simulink model "MdXX_QuitReason"  (R2018b)
settings: Solver=FixedStepDiscrete  StartTime=0.0  StopTime=10.0  FixedStep=0.01  RelTol=1e-3
undefined symbols (not defined in the file or in its folder): MdRspLocal2
settings Model: Creator=sn2xws  LastModifiedBy=sn2xws
settings Model: ModifiedHistory=|
  | 2024.12.11 V3.0.0 CR955881
  | 2025.2.24 V3.0.1 BUG 9932326 将前提条件不满足的优先级提到最高
settings DataIOCC: SaveFormat=StructureWithTime
settings OptimizationCC: DefaultParameterBehavior=Inlined  EnhancedBackFolding=on  PassReuseOutputArgsAs=Individual arguments  ZeroExternalMemoryAtStartup=off  ZeroInternalMemoryAtStartup=off  OptimizeBlockOrder=speed  DifferentSizesBufferReuse=on  OptimizationCustomize=off
settings DebuggingCC: ParameterTunabilityLossMsg=error
settings SFSimCC: MATLABDynamicMemAlloc=off
settings RTWCC: SystemTargetFile=autosar.tlc  GenCodeOnly=on  TemplateMakefile=ert_default_tmf  Description=AUTOSAR  GenerateReport=on  IncludeHyperlinkInReport=on  LaunchReport=on  GenerateTraceInfo=on  GenerateTraceReport=on  GenerateTraceReportSl=on  GenerateTraceReportSf=on  GenerateTraceReportEml=on  GenerateCodeMetricsReport=on
settings CodeAppCC: ForceParamTrailComments=on  IgnoreCustomStorageClasses=off  OperatorAnnotations=on  SimulinkDataObjDesc=on  SFDataObjDesc=on  InsertBlockDesc=on
settings STFCustomTargetCC: TargetLangStandard=C99 (ISO)  MultiwordLength=256  ParMdlRefBuildCompliant=on  CompOptLevelCompliant=on  IncludeMdlTerminateFcn=off  CombineOutputUpdateFcns=on  SuppressErrorStatus=on  ERTCustomFileBanners=on  SupportNonFinite=off  SupportComplex=off  SupportContinuousTime=off  SupportNonInlinedSFcns=off  RemoveResetFunc=on  MATLABClassNameForMDSCustomization=Simulink.SoftwareTarget.ERTCustomization  AutosarCompliant=on  UseToolchainInfoCompliant=on  LookupTableObjectStructAxisOrder=2,1,3,4,...  LUTObjectStructOrderEvenSpacing=Size,Table,Breakpoints  SystemTargetFile=autosar.tlc
settings ERTTargetCC: TargetLangStandard=C99 (ISO)  ConcurrentExecutionCompliant=off  IncludeMdlTerminateFcn=off  SuppressErrorStatus=on  SupportNonFinite=off  SupportComplex=off  ModelStepFunctionPrototypeControlCompliant=off  CPPClassGenCompliant=off  AutosarCompliant=on  LookupTableObjectStructAxisOrder=2,1,3,4,...  LUTObjectStructOrderEvenSpacing=Size,Table,Breakpoints  InlinedParameterPlacement=NonHierarchical  ERTCustomFileTemplate=example_file_process.tlc  ERTFilePackagingFormat=Compact

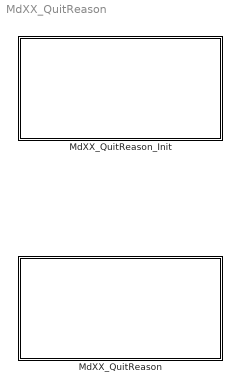
== system MdXX_QuitReason ==
  MdXX_QuitReason : Subsystem
  MdXX_QuitReason_Init : Subsystem

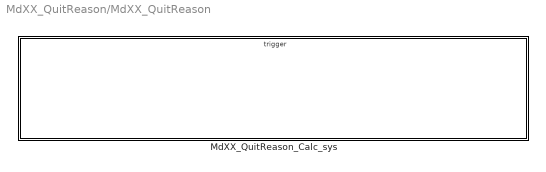
== system MdXX_QuitReason/MdXX_QuitReason ==
  MdXX_QuitReason_Calc_sys : Subsystem

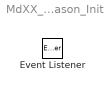
== system MdXX_QuitReason/MdXX_QuitReason_Init ==
  Event Listener : EventListener  EventName=reset

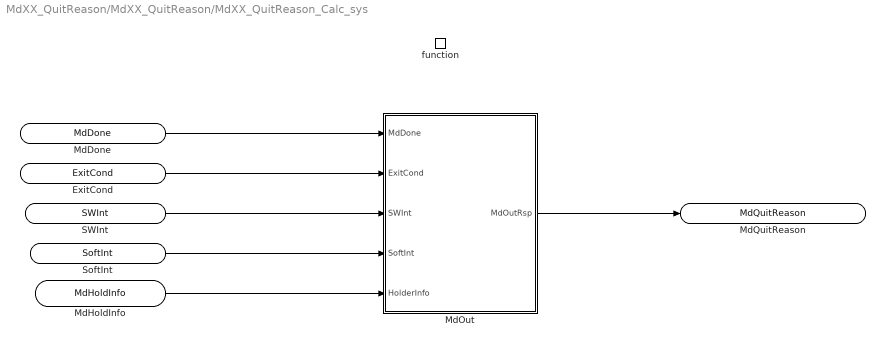
== system MdXX_QuitReason/MdXX_QuitReason/MdXX_QuitReason_Calc_sys ==
  function : TriggerPort  TriggerType=function-call  IsSimulinkFunction=on  FunctionName=MdXX_QuitReason_Calc  VariantControl=(inherit)
  MdOut : Subsystem  TreatAsAtomicUnit=on  RTWFcnName=MdRspChk
      settings: RTWFcnNameOpts=User specified
  MdDone : ArgIn  OutDataTypeStr=uint8  ArgumentName=MdDone
  ExitCond : ArgIn  Port=2  OutDataTypeStr=boolean  ArgumentName=ExitCond
  SWInt : ArgIn  Port=3  OutDataTypeStr=boolean  ArgumentName=SWInt
  SoftInt : ArgIn  Port=4  OutDataTypeStr=boolean  ArgumentName=SoftInt
  MdHoldInfo : ArgIn  Port=5  OutDataTypeStr=boolean  ArgumentName=MdHoldInfo
  MdQuitReason : ArgOut  OutDataTypeStr=Enum: MdRspLocal2  ArgumentName=MdQuitReason
  wires:
  MdDone/1 -> MdOut/1(MdDone)
  ExitCond/1 -> MdOut/2(ExitCond)
  SWInt/1 -> MdOut/3(SWInt)
  SoftInt/1 -> MdOut/4(SoftInt)
  MdOut/1(MdOutRsp) -> MdQuitReason/1
  MdHoldInfo/1 -> MdOut/5(HolderInfo)

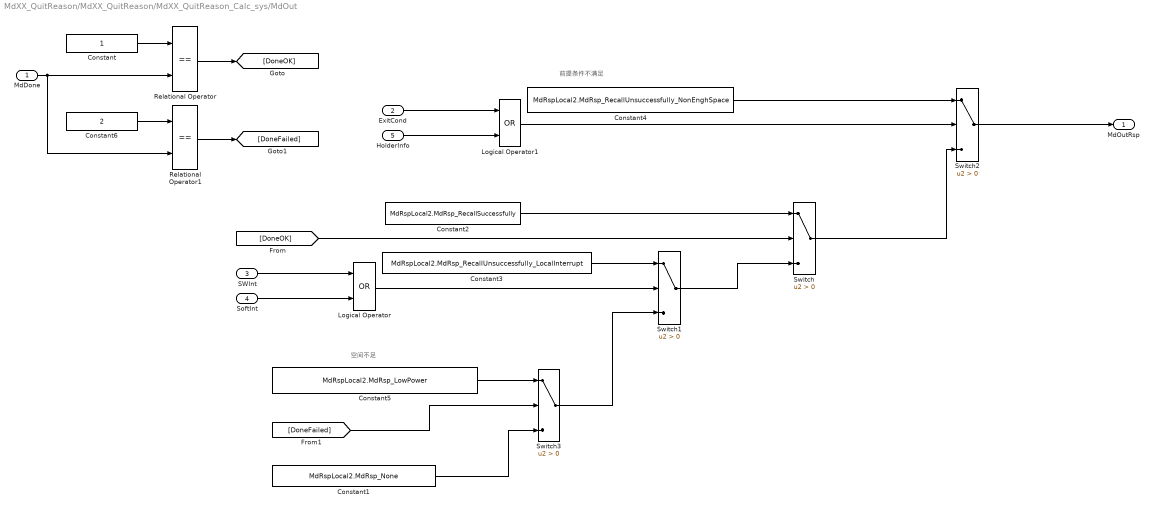
== system MdXX_QuitReason/MdXX_QuitReason/MdXX_QuitReason_Calc_sys/MdOut ==
  note: 前提条件不满足
  note: 空间不足
  MdDone : Inport
  ExitCond : Inport  Port=2
  SWInt : Inport  Port=3
  SoftInt : Inport  Port=4
  HolderInfo : Inport  Port=5
  Constant : Constant
  Constant1 : Constant  Value=MdRspLocal2.MdRsp_None  OutDataTypeStr=Enum:MdRspLocal2
  Constant2 : Constant  Value=MdRspLocal2.MdRsp_RecallSuccessfully  OutDataTypeStr=Enum:MdRspLocal2
  Constant3 : Constant  Value=MdRspLocal2.MdRsp_RecallUnsuccessfully_LocalInterrupt  OutDataTypeStr=Enum:MdRspLocal2
  Constant4 : Constant  Value=MdRspLocal2.MdRsp_RecallUnsuccessfully_NonEnghSpace  OutDataTypeStr=Enum:MdRspLocal2
  Constant5 : Constant  Value=MdRspLocal2.MdRsp_LowPower  OutDataTypeStr=Enum:MdRspLocal2
  Constant6 : Constant  Value=2
  Logical Operator : Logic  Operator=OR  AllPortsSameDT=off  OutDataTypeStr=boolean
  Logical Operator1 : Logic  Operator=OR  AllPortsSameDT=off  OutDataTypeStr=boolean
  Relational Operator : RelationalOperator  Operator===  OutDataTypeStr=boolean  RndMeth=Simplest
  Relational Operator1 : RelationalOperator  Operator===  OutDataTypeStr=boolean  RndMeth=Simplest
  Switch{,1..3} (4 alike) : Switch  Criteria=u2 > Threshold
  MdOutRsp : Outport
  wires:
  Constant4/1 -> Switch2/1
  Logical Operator/1 -> Switch1/2
  Constant3/1 -> Switch1/1
  Switch1/1 -> Switch/3
  Constant2/1 -> Switch/1
  SoftInt/1 -> Logical Operator/2
  SWInt/1 -> Logical Operator/1
  Logical Operator1/1 -> Switch2/2
  ExitCond/1 -> Logical Operator1/1
  Constant/1 -> Relational Operator/1
  MdDone/1 -> Relational Operator1/2, Relational Operator/2
  Constant6/1 -> Relational Operator1/1
  Relational Operator/1 -> [DoneOK]
  Relational Operator1/1 -> [DoneFailed]
  [DoneOK] -> Switch/2
  HolderInfo/1 -> Logical Operator1/2
  Constant1/1 -> Switch3/3
  [DoneFailed] -> Switch3/2
  Constant5/1 -> Switch3/1
  Switch/1 -> Switch2/3
  Switch2/1 -> MdOutRsp/1
  Switch3/1 -> Switch1/3
